simulink model "operational_space_control_test"  (R2024b)
settings: Solver=ode1  StartTime=0.0  StopTime=10  FixedStep=dt  RelTol=1e-3
model workspace (MAT data in the model file):
  dt = 0.001
undefined symbols (not defined in the file or in its folder): eul2tform, trvec2tform
libraries: sdu_controllers x7, robotcorelib x2
settings Model: Creator=eld  LastModifiedBy=eld

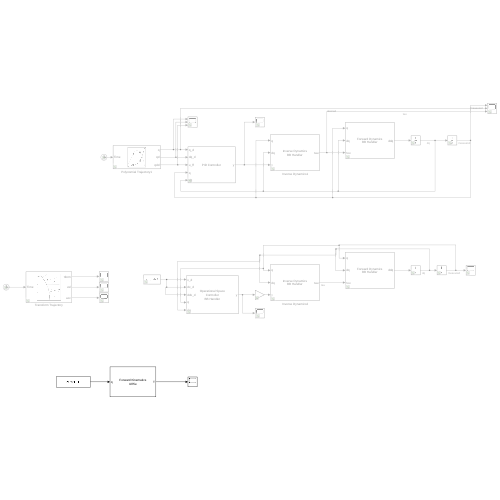
[thumbnail: Simulink's stored preview of the top-level diagram]
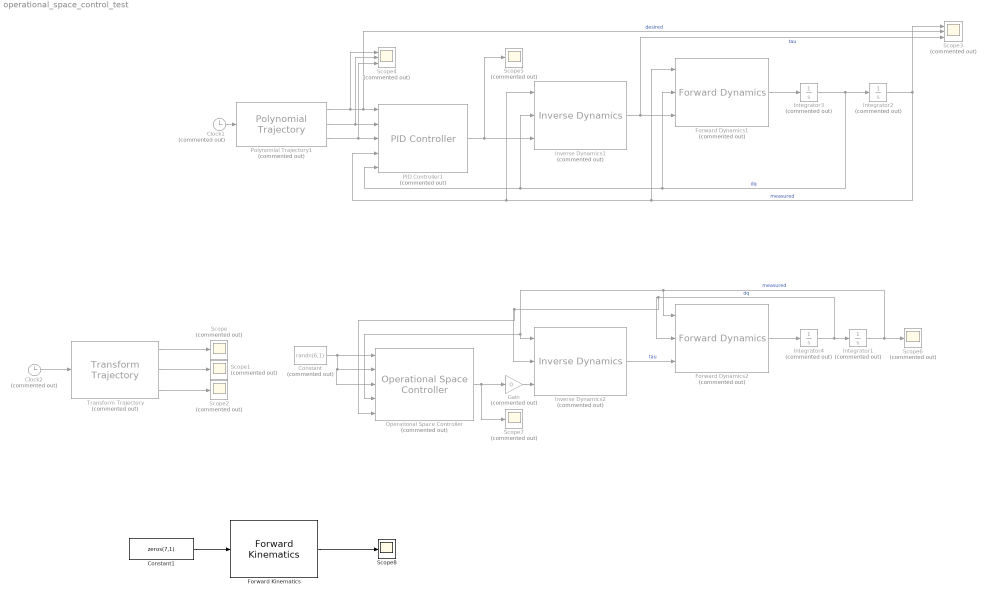
== system operational_space_control_test ==
  " Inverse Dynamics1" : sdu_controllers/Dynamics/Inverse Dynamics  Commented=on  RobotType=BB Handler  SimulateUsing=Interpreted execution
  " Inverse Dynamics2" : sdu_controllers/Dynamics/Inverse Dynamics  Commented=on  RobotType=BB Handler  SimulateUsing=Interpreted execution
  Clock1 : Clock  Commented=on
  Clock2 : Clock  Commented=on
  Constant : Constant  Commented=on  Value=randn(6,1)
  Constant1 : Constant  Value=zeros(7,1)
  Forward Dynamics1 : sdu_controllers/Dynamics/Forward Dynamics  Commented=on  RobotType=BB Handler  SimulateUsing=Interpreted execution
  Forward Dynamics2 : sdu_controllers/Dynamics/Forward Dynamics  Commented=on  RobotType=BB Handler  SimulateUsing=Interpreted execution
  Forward Kinematics : sdu_controllers/Kinematics/Forward Kinematics  RobotType=UR5e  SimulateUsing=Interpreted execution
  Gain : Gain  Commented=on  Gain=0
  Integrator1 : Integrator  Commented=on  InitialCondition=zeros(7,1)
  Integrator2 : Integrator  Commented=on  InitialCondition=[0;-pi/2;-pi/2;-pi/2;pi/2;0; 0]
  Integrator3 : Integrator  Commented=on  InitialCondition=zeros(7,1)
  Integrator4 : Integrator  Commented=on  InitialCondition=zeros(7,1)
  Operational Space Controller : sdu_controllers/Controllers/Operational Space Controller  Commented=on  Kp=eye( 7)  Kd=eye( 7)  RobotType=BB Handler  SimulateUsing=Interpreted execution
  PID Controller1 : sdu_controllers/Controllers/PID Controller  Commented=on  Kp=100.0  Ki=20  Kd=2 * sqrt( 100.0 )  N=1  num_states=6  sample_time=1 / 500.  SimulateUsing=Interpreted execution
  Polynomial Trajectory1 : robotcorelib/Polynomial Trajectory  Commented=on  WaypointSource=Internal  Waypoints="[0, -pi/2, -pi/2, -pi/2, pi/2, 0, 0;  deg2rad(45), deg2rad(-120), -pi/2, deg2rad(-60), pi/2, deg2rad(-45), 1; -1, pi/2, pi/2, pi/2, -pi/2, 1, 2].'"  TimePoints=[ 0, 25, 50]  TimeInterval=[ 1, 4 ]  Method=Quintic Polynomial  ParameterSource=Internal  VelocityBoundaryCondition=zeros( 7, 3)  AccelerationBoundaryCondition=zeros( 7,3)  SimulateUsing=Code generation
  Scope{,1..2,5..7} (6 alike) : Scope  Commented=on
  Scope3 : Scope  Commented=on  NumInputPorts=3
  Scope4 : Scope  Commented=on  NumInputPorts=3
  Scope8 : Scope
  Transform Trajectory : robotcorelib/Transform Trajectory  Commented=on  WaypointSource=Internal  T0=trvec2tform( [ 1, 10, -1 ] )  TF=eul2tform( [ 0, pi, pi / 2 ] )  TimeInterval=[ 2, 3 ]  CustomTimeScaling=off  ParameterSource=Internal  TSTime=2:0.1:3  TimeScaling=[ 0:0.1:1; ones( 1, 11 ); zeros( 1, 11 ) ]  SimulateUsing=Interpreted execution
      settings: LibrarySourceBlock=robotutilslib/Transform Trajectory
  wires:
  " Inverse Dynamics1"/1 -> Scope3/3, Forward Dynamics1/3  "tau"
  Polynomial Trajectory1/2 -> Scope4/2, PID Controller1/2
  PID Controller1/1 -> Scope5/1, " Inverse Dynamics1"/3
  Polynomial Trajectory1/3 -> Scope4/3, PID Controller1/3
  Polynomial Trajectory1/1 -> Scope4/1, Scope3/2, PID Controller1/1  "desired"
  Integrator2/1 -> Scope3/1, PID Controller1/4, " Inverse Dynamics1"/1, Forward Dynamics1/1  "measured"
  Integrator3/1 -> Integrator2/1, PID Controller1/5, " Inverse Dynamics1"/2, Forward Dynamics1/2  "dq"
  Forward Dynamics1/1 -> Integrator3/1
  Clock1/1 -> Polynomial Trajectory1/1
  Operational Space Controller/1 -> Scope7/1, Gain/1
  Forward Dynamics2/1 -> Integrator4/1
  Integrator4/1 -> Operational Space Controller/5, " Inverse Dynamics2"/2, Forward Dynamics2/2, Integrator1/1  "dq"
  Integrator1/1 -> Scope6/1, Operational Space Controller/4, " Inverse Dynamics2"/1, Forward Dynamics2/1  "measured"
  " Inverse Dynamics2"/1 -> Forward Dynamics2/3  "tau"
  Clock2/1 -> Transform Trajectory/1
  Transform Trajectory/1 -> Scope/1
  Transform Trajectory/2 -> Scope1/1
  Transform Trajectory/3 -> Scope2/1
  Constant/1 -> Operational Space Controller/1, Operational Space Controller/3, Operational Space Controller/2
  Gain/1 -> " Inverse Dynamics2"/3
  Constant1/1 -> Forward Kinematics/1
  Forward Kinematics/1 -> Scope8/1
